simulink model "MG_Damping"  (R2020b)
settings: Solver=ode45  StartTime=0.0  StopTime=TFinal  FixedStep=0.01  RelTol=1e-6
undefined symbols (not defined in the file or in its folder): coupling, decay_rate, n, S, sample_time
libraries: simrfV2util1 x3, simrfV2elements x3, simrfV2_lib x1
settings Model: Creator=tian  LastModifiedBy=tian

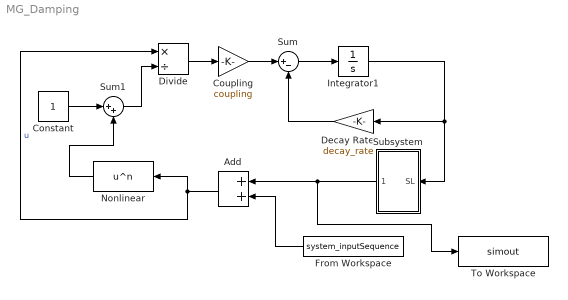
== system MG_Damping ==
  Add : Sum
  Constant : Constant
  Coupling : Gain  Gain=coupling
      mask Display: fprintf("%c", 946)
  "Decay Rate " : Gain  Gain=decay_rate
      mask Display: fprintf("%c", 947)
  Divide : Product  Inputs=*/
  From Workspace : FromWorkspace  VariableName=system_inputSequence
  Integrator1 : Integrator  IgnoreLimit=on
  Nonlinear : Fcn  Expr=u^n
  Subsystem : Subsystem
  Sum : Sum  Inputs=|+-
  Sum1 : Sum  Inputs=|++
  To Workspace : ToWorkspace  VariableName=simout  SampleTime=sample_time
  wires:
  Divide/1 -> Coupling/1
  Constant/1 -> Sum1/1
  Sum/1 -> Integrator1/1
  Integrator1/1 -> "Decay Rate "/1, Subsystem/1(SL)
  Nonlinear/1 -> Sum1/2
  Sum1/1 -> Divide/2
  "Decay Rate "/1 -> Sum/2
  Add/1 -> Divide/1, Nonlinear/1  "u"
  Coupling/1 -> Sum/1
  From Workspace/1 -> Add/2
  Subsystem/1(SL1) -> To Workspace/1, Add/1

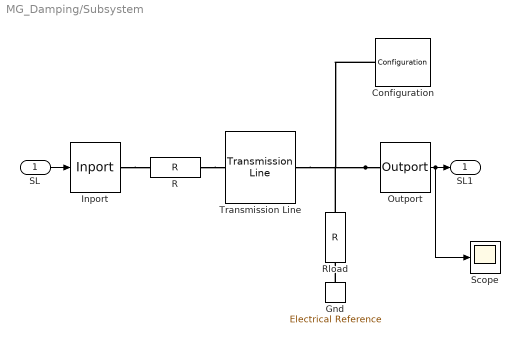
== system MG_Damping/Subsystem ==
  SL : Inport
  Configuration : simrfV2util1/Configuration  AutoFreq=on  Tones=[0] Hz  Harmonics=[1]  NormalizeCarrierPower=on  SolverType=Auto  UseCCode=on  StepSize=0.06/100 s  AddNoise=on  defaultRNG=on  Seed=0  Temperature=290 K  SolverDelFlag=0  AbsTol=1e-6  RelTol=1e-3  MaxIter=10  ErrorEstimationType=2-norm over all variables  EnableInterpFilter=on  HiddenFIRfilterControllerParam=on  SmallSignalApprox=off  AllSimFreqs=on  SimFreqs=[] Hz  SimFreqsInternal=[]  SamplesPerFrame=1
      settings: SourceProductBaseCode=RB
  Gnd : simrfV2_lib/Elements/Electrical Reference
      settings: SourceProductBaseCode=RB  InternalSimscapePortConfiguration="{\"Bottom\":[],\"Left\":[{\"id\":\"V\",\"label\":\"\",\"type\":\"foundation.rf.circuitenvelope\"}],\"Right\":[],\"Top\":[]}"
  Inport : simrfV2util1/Inport  SimulinkInputSignalType=Ideal voltage  CarrierFreq=0 Hz  ZS=0  InternalGrounding=on
      settings: SourceProductBaseCode=RB
  Outport : simrfV2util1/Outport  SensorType=Ideal voltage  OutputFormat=Real Passband  CarrierFreq=0 Hz  ZL=Inf  InternalGrounding=on  StepSize=1e-06 s  AutoStep=on
      settings: SourceProductBaseCode=RB
  R : simrfV2elements/R  classname=resistor  Resistance=5 Ohm  AddNoise=on
      settings: SourceProductBaseCode=RB
  Rload : simrfV2elements/R  classname=resistor  Resistance=10 Ohm  AddNoise=on
      settings: SourceProductBaseCode=RB
  Scope : Scope
  Transmission Line : simrfV2elements/Transmission Line  classname=xline  Model_type=Delay-based and lossy  Parameterization=By inductance and capacitance  TransDelay=0.06 s  CharImped=135 Ohm  Resistance=10 Ohm/m  Inductance=235e-9 H/m  Capacitance=94e-12 F/m  Conductance=5e-6 S/m  LineLength=1 m  NumSegments=1  InternalGrounding=on  OuterRadius=2.57 mm  InnerRadius=0.725 mm  MuR=1  EpsilonR=2.2  LossTangent=0  SigmaCond=inf S/m  StubMode=Not a stub  Termination=Open  ConductorWidth=0.6 mm  SlotWidth=0.2 mm  Height=0.635 mm  Thickness=5 um  SWidth=0.6 mm  Radius=0.67 mm  Separation=1.62 mm  PWidth=5 mm  PSeparation=1 mm  PV=299792458  Loss=1  SourceFreq=User-specified  PlotFreq=[1e9:1e6:3e9] Hz  PlotType=X-Y plane  YParam1=S(1,1)  YFormat1=Magnitude (decibels)  YParam2=S(2,2)  YFormat2=Magnitude (decibels)  YOption=Linear  XOption=Linear  FitOpt=Share all poles  FitTol=-40  SparamRepresentation=Frequency domain  Freq=1e9 Hz  Interp_type=Linear  AutoImpulseLength=off  ImpulseLength=0 s  MagModeling=off
      settings: SourceProductBaseCode=RB
  SL1 : Outport
  wires:
  Outport/1 -> Scope/1, SL1/1
  SL/1 -> Inport/1
  connections:
  Inport/RConn1 -- R/LConn1
  R/RConn1 -- Transmission Line/LConn1
  Gnd/LConn1 -- Rload/LConn1
  Outport/LConn1 -- Transmission Line/RConn1 -- Configuration/LConn1 -- Rload/RConn1
